simulink model "hiddenmessage"  (R2015b)
settings: Solver=VariableStepAuto  StartTime=0.0  StopTime=10.0  RelTol=1e-3
libraries: dspvision x2, dspadpt3 x1, dspsnks4 x1
settings Model: Creator=User  LastModifiedBy=User

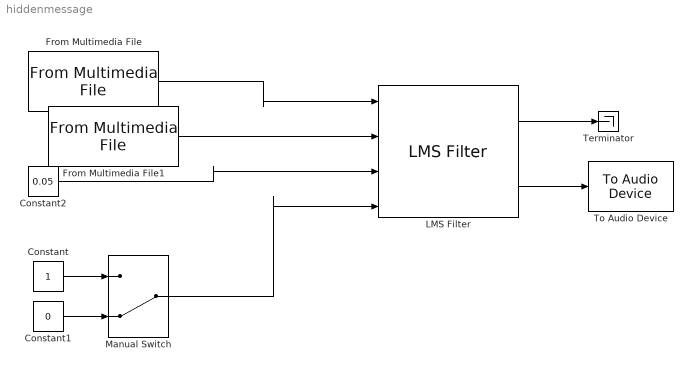
== system hiddenmessage ==
  Constant : Constant
  Constant1 : Constant  Value=0
  Constant2 : Constant  Value=0.05
  From Multimedia File : dspvision/From Multimedia File  inputFilename=C:\Users\User\Documents\Martin\EEE\second year\project\adaptivefilter1.5\messy.wav  loop=on  numPlays=inf  outputStreams=Audio only  videoDataType=single  audioDataType=double  inheritSampleTime=on  userDefinedSampleTime=1/30  noAudioOutput=off  isIntensityVideo=off  fourcc=RGB  colorVideoFormat=Separate color signals  outputEOF=off  dataOrg=Column-major  audioFrameSize=1024  computeAudioFrameSize=off  outSamplingMode=Sample based
  From Multimedia File1 : dspvision/From Multimedia File  inputFilename=C:\Users\User\Documents\Martin\EEE\second year\project\adaptivefilter1.5\noise.wav  loop=on  numPlays=inf  outputStreams=Audio only  videoDataType=single  audioDataType=double  inheritSampleTime=on  userDefinedSampleTime=1/30  noAudioOutput=off  isIntensityVideo=off  fourcc=RGB  colorVideoFormat=Separate color signals  outputEOF=off  dataOrg=Column-major  audioFrameSize=1024  computeAudioFrameSize=off  outSamplingMode=Sample based
  LMS Filter : dspadpt3/LMS Filter  Algo=Normalized LMS  L=32  stepflag=Input port  mu=0.1  leakage=1.0  ic=0  Adapt=on  resetflag=None  weights=off  secondCoeffMode=User-defined  secondCoeffWordLength=2  secondCoeffFracLength=15  accum2Mode=User-defined  accum2FracLength=20  prodOutput2Mode=User-defined  prodOutput2FracLength=20  prodOutput3Mode=User-defined  prodOutput3FracLength=20  prodOutput4Mode=User-defined  prodOutput4FracLength=20  quotientMode=User-defined  quotientFracLength=20  roundingMode=Floor  overflowMode=off  addnparflag=off
  Manual Switch : ManualSwitch  CurrentSetting=0
  Terminator : Terminator
  To Audio Device : dspsnks4/To Audio Device  deviceName=Default  inheritSampleRate=on  sampleRate=44100  deviceDatatype=Determine from input data type  autoBufferSize=on  bufferSize=4096  queueDuration=1.0  defaultOutputChannelMapping=on  outputChannelMapping=1:2  outputNumUnderrunSamples=off
  wires:
  From Multimedia File/1 -> LMS Filter/1
  Manual Switch/1 -> LMS Filter/4
  Constant1/1 -> Manual Switch/2
  Constant/1 -> Manual Switch/1
  Constant2/1 -> LMS Filter/3
  From Multimedia File1/1 -> LMS Filter/2
  LMS Filter/1 -> Terminator/1
  LMS Filter/2 -> To Audio Device/1
